simulink model "FDIlinkSimulinkSerial_2018a"  (R2022a)
settings: Solver=VariableStepAuto  StartTime=0.0  StopTime=inf  RelTol=1e-3
libraries: instrumentseriallib x2, aerolibconvert2 x1, sharedtransform x1
settings Model: Creator=JackyL  LastModifiedBy=edison
settings SolverCC: AlgebraicLoopSolver=TrustRegion
settings DataIOCC: ReturnWorkspaceOutputs=off
settings DebuggingCC: UnconnectedInputMsg=warning  UnconnectedOutputMsg=warning  UnconnectedLineMsg=warning  SFMachineParentedDataDiag=warning  ArithmeticOperatorsInVariantConditions=warning
settings SFSimCC: CustomCodeUndefinedFunction=UseInterfaceOnly
settings RTWCC: DLArmComputeVersion=19.05

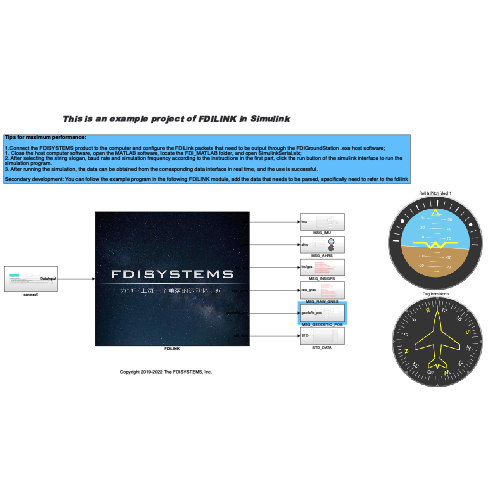
[thumbnail: Simulink's stored preview of the top-level diagram]
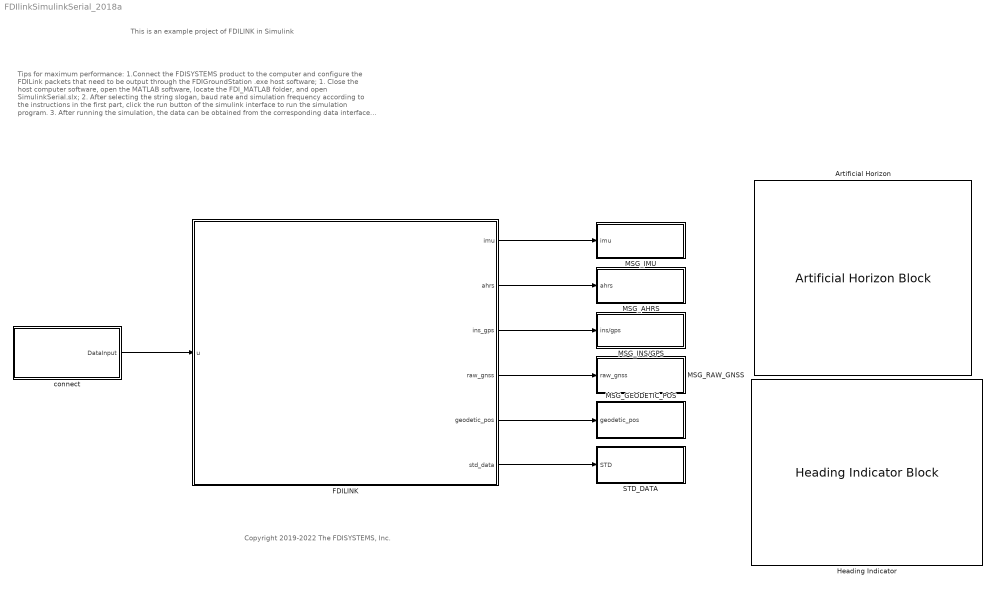
== system FDIlinkSimulinkSerial_2018a ==
  note: This is an example project of FDILINK in Simulink
  note: Copyright 2019-2022 The FDISYSTEMS, Inc.
  note: Tips for maximum performance:
      |
      | 1.Connect the FDISYSTEMS product to the computer and configure the FDILink packets that need to be output through the FDIGroundStation .exe host software;
      | 1. Close the host computer software, open the MATLAB software, locate the FDI_MATLAB folder, and open SimulinkSerial.slx;
      | 2. After selecting the string slogan, baud rate and simulation frequency according to the instructions in the first part, click the run button of the simulink interface to run the simulation program.
      | 3. After running the simulation, the data can be obtained from the corresponding data interface in real time, and the use is successful.
      |
      | Secondary development: You can follow the example program in the following FDILINK module, add the data that needs to be parsed, specifically need to refer to the fdilink protocol document to write, and finally, pay attention to the computer software to enable this data frame.
  Artificial Horizon : ArtificialHorizonBlock
  FDILINK : MATLAB Function  TreatAsAtomicUnit=on
  Heading Indicator : HeadingIndicatorBlock
  "MSG_AHRS " : Subsystem
  MSG_GEODETIC_POS : Subsystem
  "MSG_IMU " : Subsystem
  MSG_INS/GPS : Subsystem
  MSG_RAW_GNSS : Subsystem
  STD_DATA : Subsystem
  connect : Subsystem
  wires:
  connect/1(DataInput) -> FDILINK/1(u)
  FDILINK/1(imu) -> "MSG_IMU "/1("imu ")
  FDILINK/2(ahrs) -> "MSG_AHRS "/1("ahrs ")
  FDILINK/3(ins_gps) -> MSG_INS/GPS/1("ins/gps ")
  FDILINK/4(raw_gnss) -> MSG_RAW_GNSS/1("raw_gnss ")
  FDILINK/5(geodetic_pos) -> MSG_GEODETIC_POS/1("geodetic_pos ")
  FDILINK/6(std_data) -> STD_DATA/1(STD)

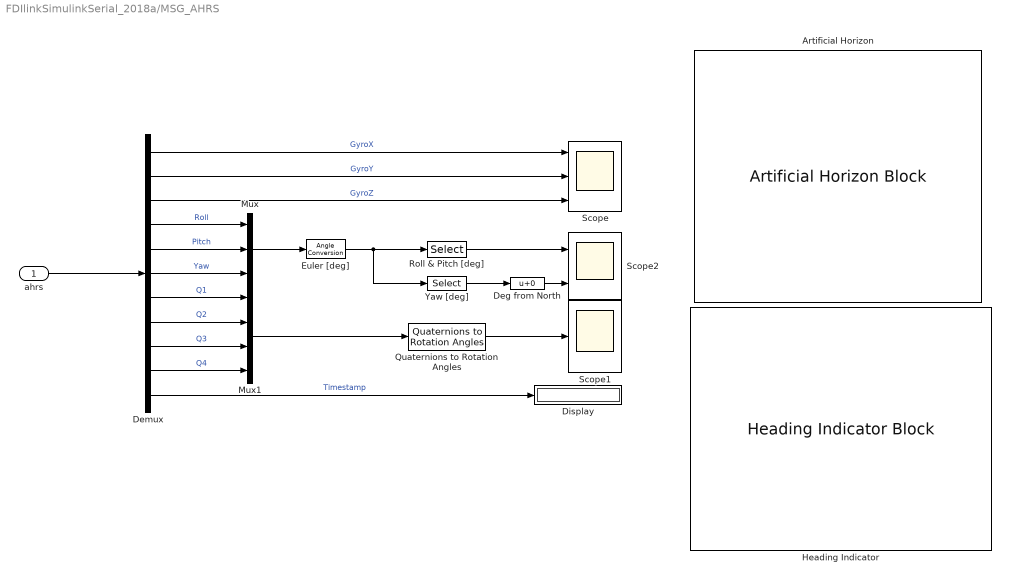
== system FDIlinkSimulinkSerial_2018a/MSG_AHRS  ==
  "ahrs " : Inport
  Artificial Horizon : ArtificialHorizonBlock
  Deg from North : Bias  SaturateOnIntegerOverflow=off
  Demux : Demux  Outputs=11
  Display : Display
  Euler [deg] : aerolibconvert2/Angle Conversion  IU=rad  OU=deg
  Heading Indicator : HeadingIndicatorBlock
  Mux : Mux  Inputs=3
  Mux1 : Mux
  Quaternions to Rotation Angles : sharedtransform/Quaternions to Rotation Angles  rotationOrder=ZYX  aMode=aMode
      settings: SourceProductBaseCode=AE,PW,DR,MT,VE
  Roll & Pitch [deg] : Selector  InputPortWidth=3  IndexOptions=Index vector (dialog)  Indices=[1 2]  OutputSizes=1
  Scope : Scope  NumInputPorts=3
  Scope1 : Scope
  Scope2 : Scope  NumInputPorts=2
  Yaw [deg] : Selector  InputPortWidth=3  IndexOptions=Index vector (dialog)  Indices=[3]  OutputSizes=1
  wires:
  "ahrs "/1 -> Demux/1
  Demux/1 -> Scope/1  "GyroX"
  Demux/2 -> Scope/2  "GyroY"
  Demux/3 -> Scope/3  "GyroZ"
  Demux/5 -> Mux/2  "Pitch"
  Demux/7 -> Mux1/1  "Q1"
  Demux/8 -> Mux1/2  "Q2"
  Demux/9 -> Mux1/3  "Q3"
  Demux/10 -> Mux1/4  "Q4"
  Demux/11 -> Display/1  "Timestamp"
  Demux/4 -> Mux/1  "Roll"
  Demux/6 -> Mux/3  "Yaw"
  Mux/1 -> Euler [deg]/1
  Euler [deg]/1 -> Yaw [deg]/1, Roll & Pitch [deg]/1
  Yaw [deg]/1 -> Deg from North/1
  Mux1/1 -> Quaternions to Rotation Angles/1
  Quaternions to Rotation Angles/1 -> Scope1/1
  Roll & Pitch [deg]/1 -> Scope2/1
  Deg from North/1 -> Scope2/2

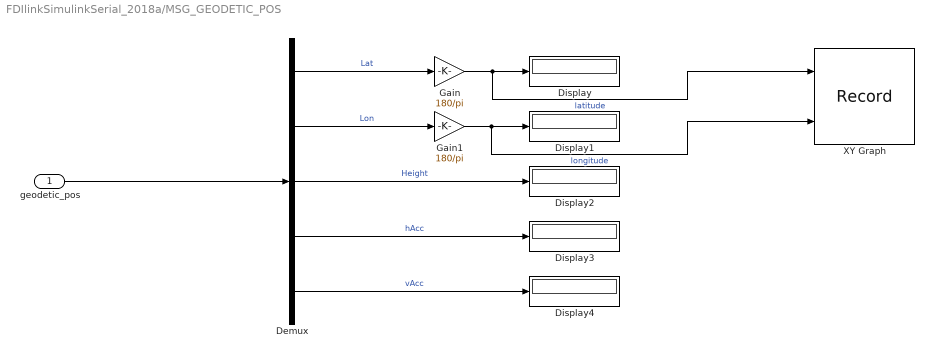
== system FDIlinkSimulinkSerial_2018a/MSG_GEODETIC_POS ==
  "geodetic_pos " : Inport
  Demux : Demux  Outputs=5
  Display{,1..4} (5 alike) : Display
  Gain : Gain  Gain=180/pi
  Gain1 : Gain  Gain=180/pi
  XY Graph : Record  FileSettingsInternal="{\"entries\":[{\"content\":{\"excelSettings\":{\"content\":{},\"type\":\"Streamout.ExcelSettings\"}},\"type\":\"Streamout.FileSettingStorage\",\"uuid\":\"a69ffe78-a3a6-46ae-8698-81ae45eb2b06\"}],\"packageUris\":[\"http://schema.mathworks.com/mf0/streamout_blocks/R2020a\"],\"version\":\"1.0\"}"  Layout=[1 1]  SignalsInternal="{\"entries\":[{\"content\":{\"signals\":[{\"content\":{\"blockPath\":[\"FDIlinkSimulinkSerial/MSG_GEODETIC_POS/XY Graph\"],\"channel\":[],\"dimensions\":[1],\"domain\":\"FDIlinkSimulinkSerial/MSG_GEODETIC_POS/XY Graph\",\"lineColor\":\"#a2142f\",\"plots\":[1],\"port\":1,\"sid\":[],\"signalID\":25,\"signalName\":\"latitude\"},\"type\":\"RecordBlkView.Signal\",\"uuid\":\"5e8f73f3-3c43-46e3-88b4-6193506b65e4\"},{\"content\":{\"blockPath\":[\"FDIlinkSimulinkSerial/MSG_GEODETIC_POS/XY Graph\"],\"channel\":[],\"dimensions\":[1],\"domain\":\"FDIlinkSimulinkSerial/MSG_GEODETIC_POS/XY Graph\",\"lineColor\":\"#139fff\",\"plots\":[1],\"port\":2,\"sid\":[],\"signalID\":28,\"signalName\":\"longitude\"},\"type\":\"RecordBlkView.Signal\",\"uuid\":\"f4642996-ede7-4ff7-91cc-e7905eb53ce7\"}]},\"type\":\"RecordBlkView.InputSignals\",\"uuid\":\"4c3864db-8a4e-40ce-a69a-83f8d065a781\"}],\"packageUris\":[\"http://schema.mathworks.com/mf0/streamout_blocks/R2020a\"],\"version\":\"1.0\"}"  VisualizationBindings="{\"mapsplugin\":{\"info\":[{\"bindingParametersList\":[{\"parameter\":\"Latitude\",\"signalID\":25,\"signalName\":\"latitude\"},{\"parameter\":\"Longitude\",\"signalID\":28,\"signalName\":\"longitude\"}],\"subplotID\":1}]}}"  CompatibilityTag=XY
  wires:
  "geodetic_pos "/1 -> Demux/1
  Demux/1 -> Gain/1  "Lat"
  Demux/3 -> Display2/1  "Height"
  Demux/4 -> Display3/1  "hAcc"
  Demux/2 -> Gain1/1  "Lon"
  Gain/1 -> XY Graph/1, Display/1  "latitude"
  Gain1/1 -> XY Graph/2, Display1/1  "longitude"
  Demux/5 -> Display4/1  "vAcc"

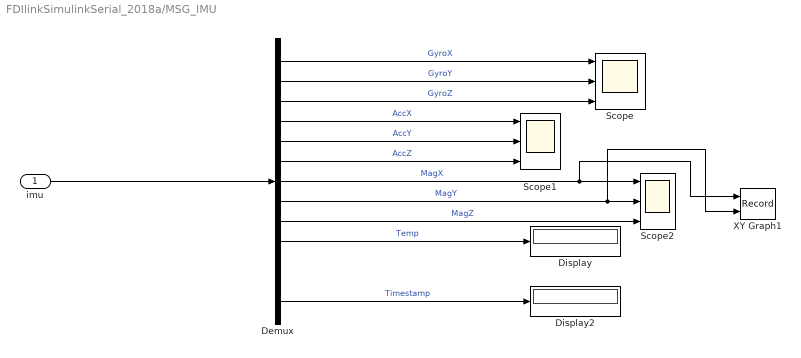
== system FDIlinkSimulinkSerial_2018a/MSG_IMU  ==
  "imu " : Inport
  Demux : Demux  Outputs=13
  Display : Display
  Display2 : Display
  Scope : Scope  NumInputPorts=3
  Scope1 : Scope  NumInputPorts=3
  Scope2 : Scope  NumInputPorts=3
  XY Graph1 : Record  FileSettingsInternal="{\"entries\":[{\"content\":{\"excelSettings\":{\"content\":{},\"type\":\"Streamout.ExcelSettings\"}},\"type\":\"Streamout.FileSettingStorage\",\"uuid\":\"11816fbf-3a81-431f-b36e-f5940fcd8774\"}],\"packageUris\":[\"http://schema.mathworks.com/mf0/streamout_blocks/R2020a\"],\"version\":\"1.0\"}"  Layout=[1 1]  SignalsInternal="{\"entries\":[{\"content\":{\"signals\":[{\"content\":{\"blockPath\":[\"FDIlinkSimulinkSerial/MSG_IMU /XY Graph1\"],\"channel\":[],\"dimensions\":[1],\"domain\":\"FDIlinkSimulinkSerial/MSG_IMU /XY Graph1\",\"lineColor\":\"#edb120\",\"plots\":[1],\"port\":1,\"sid\":[],\"signalID\":17,\"signalName\":\"MagX\"},\"type\":\"RecordBlkView.Signal\",\"uuid\":\"38ede094-791f-412e-8a66-eb45392f3306\"},{\"content\":{\"blockPath\":[\"FDIlinkSimulinkSerial/MSG_IMU /XY Graph1\"],\"channel\":[],\"dimensions\":[1],\"domain\":\"FDIlinkSimulinkSerial/MSG_IMU /XY Graph1\",\"lineColor\":\"#7e2f8e\",\"plots\":[1],\"port\":2,\"sid\":[],\"signalID\":20,\"signalName\":\"MagY\"},\"type\":\"RecordBlkView.Signal\",\"uuid\":\"0b0ce370-550e-4cca-a288-e2ad5ff04095\"}]},\"type\":\"RecordBlkView.InputSignals\",\"uuid\":\"e286a908-9618-4894-8b76-9b35e5f09ec6\"}],\"packageUris\":[\"http://schema.mathworks.com/mf0/streamout_blocks/R2020a\"],\"version\":\"1.0\"}"  VisualizationBindings="{\"xyplotplugin\":{\"info\":[{\"series\":[{\"bindingParametersList\":[{\"parameter\":\"Y-Axis\",\"signalID\":20,\"signalName\":\"MagY\"},{\"parameter\":\"X-Axis\",\"signalID\":17,\"signalName\":\"MagX\"}],\"seriesID\":5324}],\"subplotID\":1}]}}"  CompatibilityTag=XY
  wires:
  "imu "/1 -> Demux/1
  Demux/2 -> Scope/2  "GyroY"
  Demux/10 -> Display/1  "Temp"
  Demux/8 -> XY Graph1/2, Scope2/2  "MagY"
  Demux/5 -> Scope1/2  "AccY"
  Demux/7 -> XY Graph1/1, Scope2/1  "MagX"
  Demux/6 -> Scope1/3  "AccZ"
  Demux/9 -> Scope2/3  "MagZ"
  Demux/3 -> Scope/3  "GyroZ"
  Demux/4 -> Scope1/1  "AccX"
  Demux/1 -> Scope/1  "GyroX"
  Demux/13 -> Display2/1  "Timestamp"

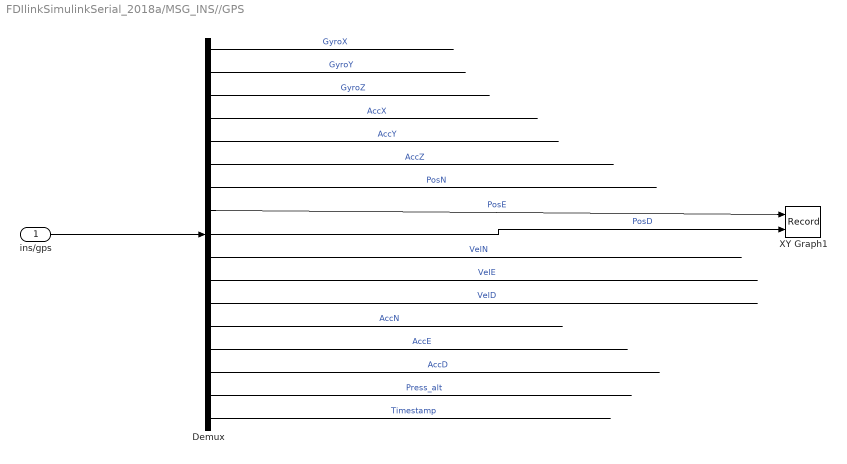
== system FDIlinkSimulinkSerial_2018a/MSG_INS//GPS ==
  "ins/gps " : Inport
  Demux : Demux  Outputs=17
  XY Graph1 : Record  FileSettingsInternal="{\"entries\":[{\"content\":{\"excelSettings\":{\"content\":{},\"type\":\"Streamout.ExcelSettings\"}},\"type\":\"Streamout.FileSettingStorage\",\"uuid\":\"ce9334ed-909b-45ed-83e3-2134e00df733\"}],\"packageUris\":[\"http://schema.mathworks.com/mf0/streamout_blocks/R2020a\"],\"version\":\"1.0\"}"  Layout=[1 1]  SignalsInternal="{\"entries\":[{\"content\":{\"signals\":[{\"content\":{\"blockPath\":[\"FDIlinkSimulinkSerial/MSG_INS//GPS/XY Graph1\"],\"channel\":[],\"dimensions\":[1],\"domain\":\"FDIlinkSimulinkSerial/MSG_INS//GPS/XY Graph1\",\"lineColor\":\"#ff13a6\",\"plots\":[1],\"port\":1,\"sid\":[],\"signalID\":9,\"signalName\":\"PosE\"},\"type\":\"RecordBlkView.Signal\",\"uuid\":\"6a2a4e0e-a427-49ba-858b-7ceb540e43af\"},{\"content\":{\"blockPath\":[\"FDIlinkSimulinkSerial/MSG_INS//GPS/XY Graph1\"],\"channel\":[],\"dimensions\":[1],\"domain\":\"FDIlinkSimulinkSerial/MSG_INS//GPS/XY Graph1\",\"lineColor\":\"#fe330a\",\"plots\":[1],\"port\":2,\"sid\":[],\"signalID\":12,\"signalName\":\"PosD\"},\"type\":\"RecordBlkView.Signal\",\"uuid\":\"6dd81a33-0683-46a8-a77b-30a409e6a004\"}]},\"type\":\"RecordBlkView.InputSignals\",\"uuid\":\"efed45c9-699c-40b8-a7df-cedaf28915f3\"}],\"packageUris\":[\"http://schema.mathworks.com/mf0/streamout_blocks/R2020a\"],\"version\":\"1.0\"}"  VisualizationBindings="{\"xyplotplugin\":{\"info\":[{\"series\":[{\"bindingParametersList\":[{\"parameter\":\"X-Axis\",\"signalID\":9,\"signalName\":\"PosE\"},{\"parameter\":\"Y-Axis\",\"signalID\":12,\"signalName\":\"PosD\"}],\"seriesID\":63831}],\"subplotID\":1}]}}"  CompatibilityTag=XY
  wires:
  "ins/gps "/1 -> Demux/1
  Demux/1 -> ?  "GyroX"
  Demux/2 -> ?  "GyroY"
  Demux/3 -> ?  "GyroZ"
  Demux/4 -> ?  "AccX"
  Demux/5 -> ?  "AccY"
  Demux/6 -> ?  "AccZ"
  Demux/7 -> ?  "PosN"
  Demux/8 -> XY Graph1/1  "PosE"
  Demux/9 -> XY Graph1/2  "PosD"
  Demux/10 -> ?  "VelN"
  Demux/11 -> ?  "VelE"
  Demux/12 -> ?  "VelD"
  Demux/13 -> ?  "AccN"
  Demux/14 -> ?  "AccE"
  Demux/15 -> ?  "AccD"
  Demux/16 -> ?  "Press_alt"
  Demux/17 -> ?  "Timestamp"

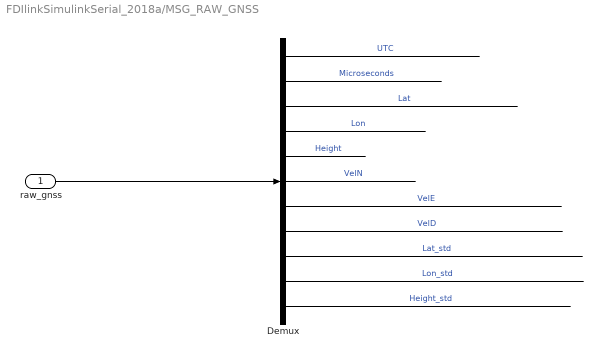
== system FDIlinkSimulinkSerial_2018a/MSG_RAW_GNSS ==
  "raw_gnss " : Inport
  Demux : Demux  Outputs=11
  wires:
  "raw_gnss "/1 -> Demux/1
  Demux/1 -> ?  "UTC"
  Demux/2 -> ?  "Microseconds"
  Demux/3 -> ?  "Lat"
  Demux/5 -> ?  "Height"
  Demux/7 -> ?  "VelE"
  Demux/8 -> ?  "VelD"
  Demux/9 -> ?  "Lat_std"
  Demux/10 -> ?  "Lon_std"
  Demux/11 -> ?  "Height_std"
  Demux/4 -> ?  "Lon"
  Demux/6 -> ?  "VelN"

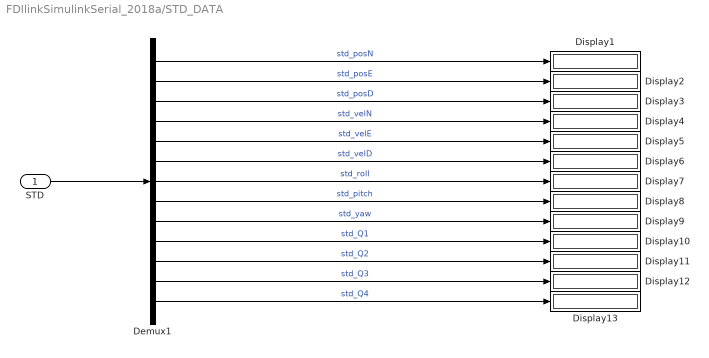
== system FDIlinkSimulinkSerial_2018a/STD_DATA ==
  STD : Inport
  Demux1 : Demux  Outputs=13
  Display{1..13} (13 alike) : Display
  wires:
  Demux1/7 -> Display7/1  "std_roll"
  Demux1/5 -> Display5/1  "std_velE"
  Demux1/4 -> Display4/1  "std_velN"
  Demux1/12 -> Display12/1  "std_Q3"
  Demux1/8 -> Display8/1  "std_pitch"
  Demux1/1 -> Display1/1  "std_posN"
  STD/1 -> Demux1/1
  Demux1/3 -> Display3/1  "std_posD"
  Demux1/6 -> Display6/1  "std_velD"
  Demux1/13 -> Display13/1  "std_Q4"
  Demux1/10 -> Display10/1  "std_Q1"
  Demux1/11 -> Display11/1  "std_Q2"
  Demux1/9 -> Display9/1  "std_yaw"
  Demux1/2 -> Display2/1  "std_posE"

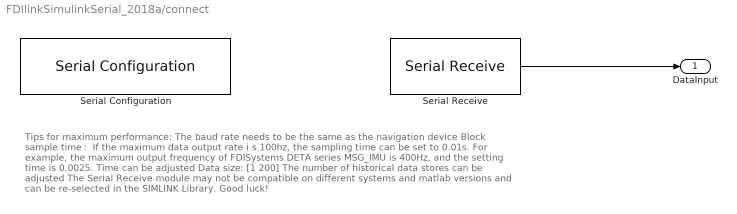
== system FDIlinkSimulinkSerial_2018a/connect ==
  note: Tips for maximum performance:
      |
      | The baud rate needs to be the same as the navigation device
      | Block sample time： If the maximum data output rate i s 100hz, the sampling time can be set to 0.01s. For example, the maximum output frequency of FDISystems DETA series MSG_IMU is 400Hz, and the setting time is 0.0025. Time can be adjusted
      | Data size：[1 200] The number of historical data stores can be adjusted
      | The Serial Receive module may not be compatible on different systems and matlab versions and can be re-selected in the SIMLINK Library. Good luck!
  Serial Configuration : instrumentseriallib/Serial Configuration  Priority=-200000  PortSel=/dev/cu.usbserial-0001  Port=/dev/cu.usbserial-0001  ComPort=/dev/cu.usbserial-0001  BaudRate=921600  DataBits=8  Parity=none  StopBits=1  ByteOrder=little-endian  FlowControl=none  Timeout=10  SimulateUsing=Interpreted execution  BlockInModel=on  aMode=1
      settings: SourceProductBaseCode=OT,IC,MT
  Serial Receive : instrumentseriallib/Serial Receive  Priority=1  PortSel=/dev/cu.usbserial-0001  Port=/dev/cu.usbserial-0001  ComPort=/dev/cu.usbserial-0001  DataType=uint8  SaveDataType=uint8  ToggleHeader=off  Header=[]  ToggleTerminator=off  Terminator=<none>  CustomTerminator=[]  InputFormat=Column major  ToggleDataSize=on  DataSize=[1 200]  EnableBlockingMode=on  ActionDataUnavailable=Output last received value  ActionWhenDataUnavailable=Output last received value  CustomValue=0  SampleTime=0.01  SimulateUsing=Interpreted execution  BlockInModel=on  aMode=1
      settings: SourceProductBaseCode=OT,IC,MT
  DataInput : Outport
  wires:
  Serial Receive/1 -> DataInput/1

== matlab function FDIlinkSimulinkSerial_2018a/FDILINK ==
  data: imu output; u input; ahrs output; ins_gps output; raw_gnss output; geodetic_pos output; std_data output
%% Describes decoding FDILink communication protocol data frames in MATLAB & simulink
% You can follow the example program in the following FDILINK module, 
% add the data that needs to be parsed, specifically need to refer to the fdilink protocol document to write, 
% and finally, pay attention to the computer software to enable this data frame.

% Copyright 2019-2021 The FDISYSTEMS, Inc.

function [imu,ahrs,ins_gps,raw_gnss,geodetic_pos,std_data] = fcn(u)
persistent FStatus;   
persistent ReceiveDataLeft;
persistent ReceiveType;
persistent Buffer;
persistent BufferIndex;
persistent lastImu;
persistent lastAhrs;
persistent lastInsGps;
persistent lastRawGnss;
persistent lastGeodeticPos;
persistent lastStdData;
if isempty(FStatus)
	FStatus = 0;
	ReceiveDataLeft = uint8(0);
	BufferIndex = uint8(0);
	Buffer = uint8(zeros(1,256));
	ReceiveType = uint8(0);
	lastImu  = zeros(13,1);
    lastAhrs = zeros(11,1);
    lastInsGps = zeros(17,1);
    lastRawGnss = zeros(11,1);
    lastGeodeticPos = zeros(5,1);
    lastStdData = zeros(13,1);
end
%数据帧帧头FC
SerialBoot_STX_Flag = uint8(252);
%数据帧帧尾FD
SerialBoot_EDX_Flag = uint8(253);
for i = 1:length(u)
	value = u(i);
	switch (FStatus)
		case 0
			ReceiveDataLeft = uint8(0);
			if value == SerialBoot_STX_Flag
				FStatus = 1;
			end
		case 1
        %ReceiveType对应数据帧里的指令类别，比如IMU数据包为0x40，AHRS数据包为0x41，转化为十进制就是64和65；
			ReceiveType = value;
			FStatus = 2;
		case 2
        %ReceiveDataLeft对应数据帧里的暂未复制带Buffer里的数据长度（位），此时被赋予的值对应该数据包完整的数据长度；
			ReceiveDataLeft = value;
			BufferIndex = uint8(1);
			FStatus = 3;
		case 3
			FStatus = 4;
		case 4
			if ReceiveDataLeft == 0
				FStatus = 0;
			else
				FStatus = 5;
			end
		case 5
			FStatus = 6;
		case 6
			FStatus = 7;
		case 7
        %对应数据帧里的载荷，此时Buffer数据按顺序存储载荷里的数据直到全部复制完成
			Buffer(BufferIndex) = value;
			BufferIndex = BufferIndex + 1;
			ReceiveDataLeft = ReceiveDataLeft - 1;
			if ReceiveDataLeft == 0
				FStatus = 8;
			end
		case 8
			if (value == SerialBoot_EDX_Flag)
				switch(ReceiveType)
					case 64
						%% 解析MSG_IMU
						lastImu(1) = typecast(Buffer(1:4),'single');
						lastImu(2) = typecast(Buffer(5:8),'single');
						lastImu(3) = typecast(Buffer(9:12),'single');
						lastImu(4) = typecast(Buffer(13:16),'single');
						lastImu(5) = typecast(Buffer(17:20),'single');
						lastImu(6) = typecast(Buffer(21:24),'single');
						lastImu(7) = typecast(Buffer(25:28),'single');
						lastImu(8) = typecast(Buffer(29:32),'single');
						lastImu(9) = typecast(Buffer(33:36),'single');
						lastImu(10) = typecast(Buffer(37:40),'single');
						lastImu(11) = typecast(Buffer(41:44),'single');
                        lastImu(12) = typecast(Buffer(45:48),'single');
                        lastImu(13) = typecast(Buffer(49:56),'uint64');
					case 65
						%% 解析MSG_AHRS
						lastAhrs(1) = typecast(Buffer(1:4),'single');
						lastAhrs(2) = typecast(Buffer(5:8),'single');
						lastAhrs(3) = typecast(Buffer(9:12),'single');
						lastAhrs(4) = typecast(Buffer(13:16),'single');
						lastAhrs(5) = typecast(Buffer(17:20),'single');
						lastAhrs(6) = typecast(Buffer(21:24),'single');
						lastAhrs(7) = typecast(Buffer(25:28),'single');
						lastAhrs(8) = typecast(Buffer(29:32),'single');
						lastAhrs(9) = typecast(Buffer(33:36),'single');
						lastAhrs(10) = typecast(Buffer(37:40),'single');
                        lastAhrs(11) = typecast(Buffer(41:48),'uint64');
					case 66
						%% 解析MSG_INS/GPS
						lastInsGps(1) = typecast(Buffer(1:4),'single');
						lastInsGps(2) = typecast(Buffer(5:8),'single');
						lastInsGps(3) = typecast(Buffer(9:12),'single');
						lastInsGps(4) = typecast(Buffer(13:16),'single');
						lastInsGps(5) = typecast(Buffer(17:20),'single');
						lastInsGps(6) = typecast(Buffer(21:24),'single');
						lastInsGps(7) = typecast(Buffer(25:28),'single');
						lastInsGps(8) = typecast(Buffer(29:32),'single');
						lastInsGps(9) = typecast(Buffer(33:36),'single');
						lastInsGps(10) = typecast(Buffer(37:40),'single');
                        lastInsGps(11) = typecast(Buffer(41:44),'single');
                        lastInsGps(12) = typecast(Buffer(45:48),'single');
                        lastInsGps(13) = typecast(Buffer(49:52),'single');
                        lastInsGps(14) = typecast(Buffer(53:56),'single');
                        lastInsGps(15) = typecast(Buffer(57:60),'single');
                        lastInsGps(16) = typecast(Buffer(61:64),'single');
                        lastInsGps(17) = typecast(Buffer(65:72),'uint64');
					case 89
						%% 解析MSG_RAW_GNSS
						lastRawGnss(1) = typecast(Buffer(1:4),'uint32');
						lastRawGnss(2) = typecast(Buffer(5:8),'uint32');
						lastRawGnss(3) = typecast(Buffer(9:16),'double');
						lastRawGnss(4) = typecast(Buffer(17:24),'double');
						lastRawGnss(5) = typecast(Buffer(25:32),'double');
						lastRawGnss(6) = typecast(Buffer(33:36),'single');
						lastRawGnss(7) = typecast(Buffer(37:40),'single');
						lastRawGnss(8) = typecast(Buffer(41:44),'single');
						lastRawGnss(9) = typecast(Buffer(45:48),'single');
						lastRawGnss(10) = typecast(Buffer(49:52),'single');
                        lastRawGnss(11) = typecast(Buffer(53:56),'single');
					case 92
						%% 解析MSG_GEODETIC_POS
						lastGeodeticPos(1) = typecast(Buffer(1:8),'double');
						lastGeodeticPos(2) = typecast(Buffer(9:16),'double');
						lastGeodeticPos(3) = typecast(Buffer(17:24),'double');
						lastGeodeticPos(4) = typecast(Buffer(25:28),'single');
						lastGeodeticPos(5) = typecast(Buffer(29:32),'single');
                    case 84
                        %% 解析MSG_POS_STD_DEV
                        lastStdData(1) =  typecast(Buffer(1:4),'single');
                        lastStdData(2) =  typecast(Buffer(5:8),'single');
                        lastStdData(3) =  typecast(Buffer(9:12),'single');
                    case 85
                        %% 解析MSG_VEL_STD_DEV
                        lastStdData(4) =  typecast(Buffer(1:4),'single');
                        lastStdData(5) =  typecast(Buffer(5:8),'single');
                        lastStdData(6) =  typecast(Buffer(9:12),'single');
                    case 86
                        %% 解析MSG_EULER_ORIEN_STD_DEV
                        lastStdData(7) =  typecast(Buffer(1:4),'single');
                        lastStdData(8) =  typecast(Buffer(5:8),'single');
                        lastStdData(9) =  typecast(Buffer(9:12),'single');
                    case 87
                        %% 解析MSG_QUAT_ORIEN_STD_DEV
                        lastStdData(10) =  typecast(Buffer(1:4),'single');
                        lastStdData(11) =  typecast(Buffer(5:8),'single');
                        lastStdData(12) =  typecast(Buffer(9:12),'single');
                        lastStdData(13) =  typecast(Buffer(13:16),'single');
                end	
			end
			FStatus = 0;
    end 
end

imu = lastImu;
ahrs = lastAhrs;
ins_gps = lastInsGps;
raw_gnss = lastRawGnss;
geodetic_pos = lastGeodeticPos;
std_data = lastStdData;

end
